simulink library "SingleWorkstationModelLibrary"  (R2014a)
settings: Solver=ode45  StartTime=0.0  StopTime=10.0  RelTol=1e-3
undefined symbols (not defined in the file or in its folder): se_randomizeseeds
(part 3 of 3)

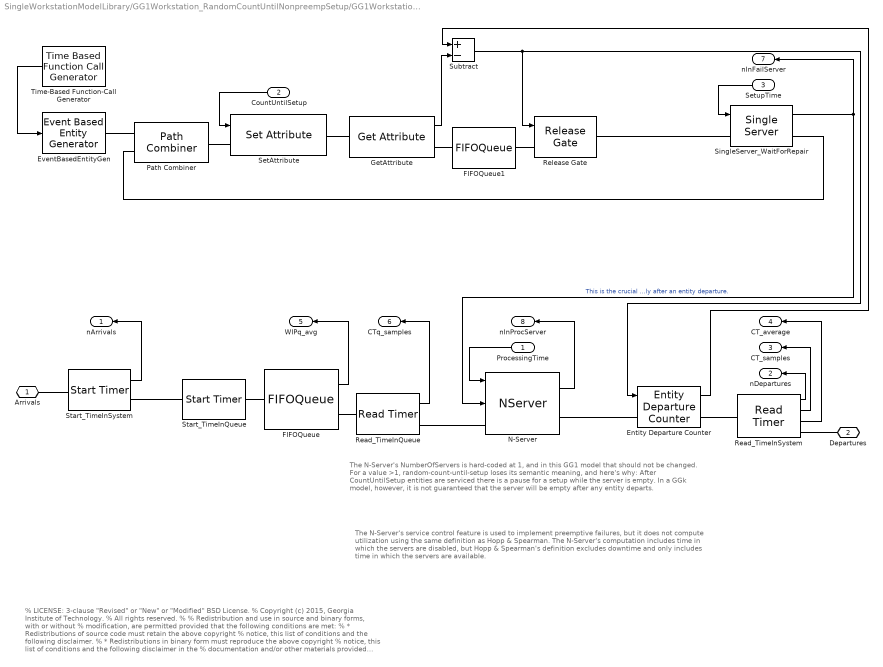
== system SingleWorkstationModelLibrary/GG1Workstation_RandomCountUntilNonpreempSetup/GG1Workstation_RandomCountUntilNonpreempSetup ==
  note: The N-Server's NumberOfServers is hard-coded at 1, and in this GG1 model that
      | should not be changed.  For a value >1, random-count-until-setup loses its semantic
      | meaning, and here's why:  After CountUntilSetup entities are serviced there is a pause
      | for a setup while the server is empty.  In a GGk model, however, it is not guaranteed
      | that the server will be empty after any entity departs.
  note: The N-Server's service control feature is used to implement preemptive failures,
      | but it does not compute utilization using the same definition as Hopp & Spearman.
      | The N-Server's computation includes time in which the servers are disabled, but
      | Hopp & Spearman's definition excludes downtime and only includes time in which
      | the servers are available.
  note: % LICENSE: 3-clause "Revised" or "New" or "Modified" BSD License.
      | % Copyright (c) 2015, Georgia Institute of Technology.
      | % All rights reserved.
      | %
      | % Redistribution and use in source and binary forms, with or without
      | % modification, are permitted provided that the following conditions are met:
      | % * Redistributions of source code must retain the above copyright
      | % notice, this list of conditions and the following disclaimer.
      | % * Redistributions in binary form must reproduce the above copyright
      | % notice, this list of conditions and the following disclaimer in the
      | % documentation and/or other materials provided with the distribution.
      | % * Neither the name of the Georgia Institute of Technology nor the
      | % names of its contributors may be used to endorse or promote products
      | % derived from this software without specific prior written permission.
      | %
      | % THIS SOFTWARE IS PROVIDED BY THE COPYRIGHT HOLDERS AND CONTRIBUTORS "AS IS" AND
      | % ANY EXPRESS OR IMPLIED WARRANTIES, INCLUDING, BUT NOT LIMITED TO, THE IMPLIED
      | % WARRANTIES OF MERCHANTABILITY AND FITNESS FOR A PARTICULAR PURPOSE ARE
      | % DISCLAIMED. IN NO EVENT SHALL THE GEORGIA INSTITUTE OF TECHNOLOGY BE LIABLE FOR
      | % ANY DIRECT, INDIRECT, INCIDENTAL, SPECIAL, EXEMPLARY, OR CONSEQUENTIAL DAMAGES
      | % (INCLUDING, BUT NOT LIMITED TO, PROCUREMENT OF SUBSTITUTE GOODS OR SERVICES;
      | % LOSS OF USE, DATA, OR PROFITS; OR BUSINESS INTERRUPTION) HOWEVER CAUSED AND
      | % ON ANY THEORY OF LIABILITY, WHETHER IN CONTRACT, STRICT LIABILITY, OR TORT
      | % (INCLUDING NEGLIGENCE OR OTHERWISE) ARISING IN ANY WAY OUT OF THE USE OF THIS
      | % SOFTWARE, EVEN IF ADVISED OF THE POSSIBILITY OF SUCH DAMAGE.
  ProcessingTime : Inport
  CountUntilSetup : Inport  Port=2
  SetupTime : Inport  Port=3
  Entity Departure Counter : EntityDepartureCounter  NumberDepartedToSignal=on  NumberDepartedToAttribute=off  CounterResetTypeOption=Trigger from port tr
  EventBasedEntityGen : EventBasedEntityGenerator  GenerateEntitiesUpon=Function call from port fcn
  FIFOQueue : FIFOQueue  Capacity=Capacity  StatAverageQueueLength=on
      settings: OutputPortMap=o3
  FIFOQueue1 : FIFOQueue  Capacity=Inf
  GetAttribute : GetAttribute  AttributeName=CountUntilSetup  EvaluatedDefaultAttributeValue={ []}
      settings: OutputPortMap=o1
  N-Server : NServer  NumberOfServers=1  ServiceTimeFrom=Signal port t  AllowServiceControl=on  BlockWhileSignalOn=on  StatNumberInBlock=on
      settings: InputPortMap=u0,u1  OutputPortMap=o1
  Path Combiner : PathCombiner  NumberInputPorts=2
  Read_TimeInQueue : ReadTimer  TimerTag=TimeInQueue  StatTimeElapsed=on
      settings: OutputPortMap=o2
  Read_TimeInSystem : ReadTimer  TimerTag=TimeInSystem  StatNumberDeparted=on  StatTimeElapsed=on  StatAverageTimeElapsed=on
      settings: OutputPortMap=o0,o2,o3
  Release Gate : ReleaseGate  OpenGateUpon=Trigger from port tr
  SetAttribute : SetAttribute  AttributeName=CountUntilSetup  AttributeFrom=Signal port  EvaluatedAttributeValue={ []}
  SingleServer_WaitForRepair : SingleServer  ServiceTimeFrom=Signal port t  AttributeName=SetupTime  StatNumberInBlock=on
      settings: OutputPortMap=o1
  Start_TimeInQueue : StartTimer  TimerTag=TimeInQueue  TimerStartedOption=Restart
  Start_TimeInSystem : StartTimer  TimerTag=TimeInSystem  TimerStartedOption=Restart  StatNumberDeparted=on
  Subtract : Sum  Inputs=+-
  Time-Based Function-Call Generator : TimeBasedFunctionCallGenerator  EventGenerationMode=Only at simulation start
  Arrivals : PMIOPort  Port=1  Side=Left
  Departures : PMIOPort  Port=2  Side=Right
  nArrivals : Outport
  nDepartures : Outport  Port=2
  CT_samples : Outport  Port=3
  CT_average : Outport  Port=4
  WIPq_avg : Outport  Port=5
  CTq_samples : Outport  Port=6
  nInFailServer : Outport  Port=7
  nInProcServer : Outport  Port=8
  wires:
  Read_TimeInSystem/2 -> CT_samples/1
  Read_TimeInQueue/1 -> CTq_samples/1
  FIFOQueue/1 -> WIPq_avg/1
  Start_TimeInSystem/1 -> nArrivals/1
  Read_TimeInSystem/1 -> nDepartures/1
  ProcessingTime/1 -> N-Server/1
  Read_TimeInSystem/3 -> CT_average/1
  Time-Based Function-Call Generator/1 -> EventBasedEntityGen/1
  CountUntilSetup/1 -> SetAttribute/1
  Subtract/1 -> Release Gate/1, Entity Departure Counter/1
  GetAttribute/1 -> Subtract/2
  Entity Departure Counter/1 -> Subtract/1
  SingleServer_WaitForRepair/1 -> nInFailServer/1, N-Server/2  "This is the crucial blocking signal - when > 0 the N-Server will be preemptively disabled. Non-preemption in this model is an approximation, because disabling of the N-Server  should follow shortly after an entity departure."
  N-Server/1 -> nInProcServer/1
  SetupTime/1 -> SingleServer_WaitForRepair/1
  connections:
  Arrivals/RConn1 -- Start_TimeInSystem/LConn1
  FIFOQueue/RConn1 -- Read_TimeInQueue/LConn1
  Start_TimeInSystem/RConn1 -- Start_TimeInQueue/LConn1
  Read_TimeInSystem/RConn1 -- Departures/RConn1
  Read_TimeInQueue/RConn1 -- N-Server/LConn1
  Start_TimeInQueue/RConn1 -- FIFOQueue/LConn1
  Path Combiner/RConn1 -- SetAttribute/LConn1
  EventBasedEntityGen/RConn1 -- Path Combiner/LConn1
  SingleServer_WaitForRepair/RConn1 -- Path Combiner/LConn2
  N-Server/RConn1 -- Entity Departure Counter/LConn1
  Entity Departure Counter/RConn1 -- Read_TimeInSystem/LConn1
  FIFOQueue1/LConn1 -- GetAttribute/RConn1
  Release Gate/RConn1 -- SingleServer_WaitForRepair/LConn1
  FIFOQueue1/RConn1 -- Release Gate/LConn1
  SetAttribute/RConn1 -- GetAttribute/LConn1

== system SingleWorkstationModelLibrary/GGkWorkstation/ComputeTH ==
  CurrentTime : Inport
  nDepartures : Inport  Port=2
  Derivative : Derivative
  Divide1 : Product  Inputs=/*
  Event to Timed Signal1 : EventToTimedSignal
  TH_average : Outport
  TH_samples : Outport  Port=2
  wires:
  CurrentTime/1 -> Divide1/1
  Event to Timed Signal1/1 -> Derivative/1, Divide1/2
  Divide1/1 -> TH_average/1
  Derivative/1 -> TH_samples/1
  nDepartures/1 -> Event to Timed Signal1/1

== system SingleWorkstationModelLibrary/GGkWorkstation/ComputeWIP ==
  nArrivals : Inport
  nDepartures : Inport  Port=2
  CurrentTime : Inport  Port=3
  Divide : Product  Inputs=*/
  Event to Timed Signal : EventToTimedSignal
  Integrator : Integrator
  Subtract : Sum  Inputs=+-
  WIP_samples : Outport
  WIP_average : Outport  Port=2
  wires:
  Subtract/1 -> WIP_samples/1, Event to Timed Signal/1
  Event to Timed Signal/1 -> Integrator/1
  Divide/1 -> WIP_average/1
  Integrator/1 -> Divide/1
  nArrivals/1 -> Subtract/1
  nDepartures/1 -> Subtract/2
  CurrentTime/1 -> Divide/2

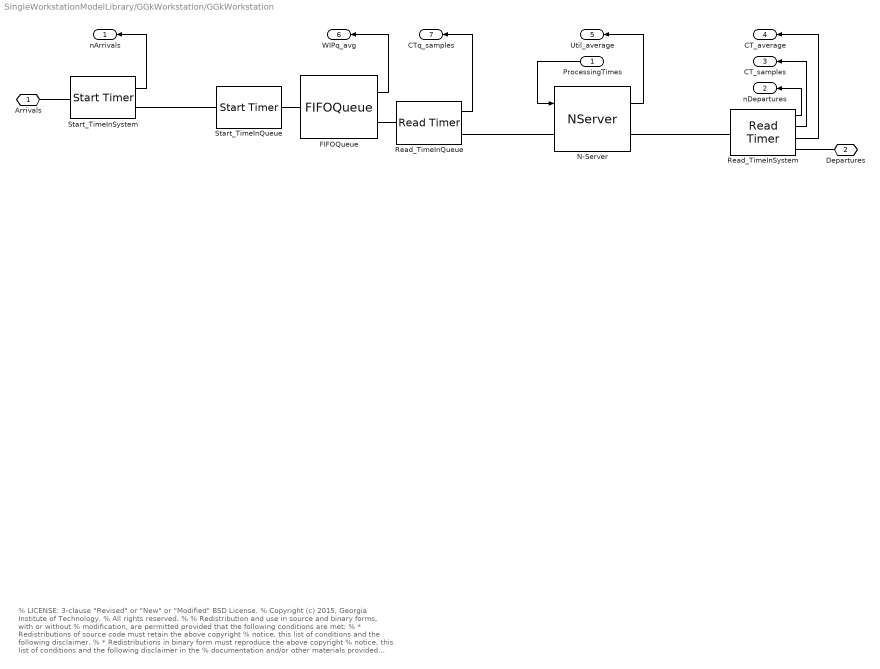
== system SingleWorkstationModelLibrary/GGkWorkstation/GGkWorkstation ==
  note: % LICENSE: 3-clause "Revised" or "New" or "Modified" BSD License.
      | % Copyright (c) 2015, Georgia Institute of Technology.
      | % All rights reserved.
      | %
      | % Redistribution and use in source and binary forms, with or without
      | % modification, are permitted provided that the following conditions are met:
      | % * Redistributions of source code must retain the above copyright
      | % notice, this list of conditions and the following disclaimer.
      | % * Redistributions in binary form must reproduce the above copyright
      | % notice, this list of conditions and the following disclaimer in the
      | % documentation and/or other materials provided with the distribution.
      | % * Neither the name of the Georgia Institute of Technology nor the
      | % names of its contributors may be used to endorse or promote products
      | % derived from this software without specific prior written permission.
      | %
      | % THIS SOFTWARE IS PROVIDED BY THE COPYRIGHT HOLDERS AND CONTRIBUTORS "AS IS" AND
      | % ANY EXPRESS OR IMPLIED WARRANTIES, INCLUDING, BUT NOT LIMITED TO, THE IMPLIED
      | % WARRANTIES OF MERCHANTABILITY AND FITNESS FOR A PARTICULAR PURPOSE ARE
      | % DISCLAIMED. IN NO EVENT SHALL THE GEORGIA INSTITUTE OF TECHNOLOGY BE LIABLE FOR
      | % ANY DIRECT, INDIRECT, INCIDENTAL, SPECIAL, EXEMPLARY, OR CONSEQUENTIAL DAMAGES
      | % (INCLUDING, BUT NOT LIMITED TO, PROCUREMENT OF SUBSTITUTE GOODS OR SERVICES;
      | % LOSS OF USE, DATA, OR PROFITS; OR BUSINESS INTERRUPTION) HOWEVER CAUSED AND
      | % ON ANY THEORY OF LIABILITY, WHETHER IN CONTRACT, STRICT LIABILITY, OR TORT
      | % (INCLUDING NEGLIGENCE OR OTHERWISE) ARISING IN ANY WAY OUT OF THE USE OF THIS
      | % SOFTWARE, EVEN IF ADVISED OF THE POSSIBILITY OF SUCH DAMAGE.
  ProcessingTimes : Inport
  FIFOQueue : FIFOQueue  Capacity=Capacity  StatAverageQueueLength=on
      settings: OutputPortMap=o3
  N-Server : NServer  NumberOfServers=NumberOfServers  ServiceTimeFrom=Signal port t  StatUtilization=on
      settings: OutputPortMap=o5
  Read_TimeInQueue : ReadTimer  TimerTag=TimeInQueue  StatTimeElapsed=on
      settings: OutputPortMap=o2
  Read_TimeInSystem : ReadTimer  TimerTag=TimeInSystem  StatNumberDeparted=on  StatTimeElapsed=on  StatAverageTimeElapsed=on
      settings: OutputPortMap=o0,o2,o3
  Start_TimeInQueue : StartTimer  TimerTag=TimeInQueue  TimerStartedOption=Restart
  Start_TimeInSystem : StartTimer  TimerTag=TimeInSystem  TimerStartedOption=Restart  StatNumberDeparted=on
  Arrivals : PMIOPort  Port=1  Side=Left
  Departures : PMIOPort  Port=2  Side=Right
  nArrivals : Outport
  nDepartures : Outport  Port=2
  CT_samples : Outport  Port=3
  CT_average : Outport  Port=4
  Util_average : Outport  Port=5
  WIPq_avg : Outport  Port=6
  CTq_samples : Outport  Port=7
  wires:
  Read_TimeInSystem/2 -> CT_samples/1
  N-Server/1 -> Util_average/1
  Read_TimeInQueue/1 -> CTq_samples/1
  FIFOQueue/1 -> WIPq_avg/1
  Start_TimeInSystem/1 -> nArrivals/1
  Read_TimeInSystem/1 -> nDepartures/1
  ProcessingTimes/1 -> N-Server/1
  Read_TimeInSystem/3 -> CT_average/1
  connections:
  Arrivals/RConn1 -- Start_TimeInSystem/LConn1
  N-Server/RConn1 -- Read_TimeInSystem/LConn1
  FIFOQueue/RConn1 -- Read_TimeInQueue/LConn1
  Start_TimeInSystem/RConn1 -- Start_TimeInQueue/LConn1
  Read_TimeInSystem/RConn1 -- Departures/RConn1
  Read_TimeInQueue/RConn1 -- N-Server/LConn1
  Start_TimeInQueue/RConn1 -- FIFOQueue/LConn1

== system SingleWorkstationModelLibrary/GGkWorkstation_MakeAndMoveBatches_Parallel/ComputeTH ==
  CurrentTime : Inport
  nDepartures : Inport  Port=2
  Derivative : Derivative
  Divide1 : Product  Inputs=/*
  Event to Timed Signal1 : EventToTimedSignal
  TH_average : Outport
  TH_samples : Outport  Port=2
  wires:
  CurrentTime/1 -> Divide1/1
  Event to Timed Signal1/1 -> Derivative/1, Divide1/2
  Divide1/1 -> TH_average/1
  Derivative/1 -> TH_samples/1
  nDepartures/1 -> Event to Timed Signal1/1

== system SingleWorkstationModelLibrary/GGkWorkstation_MakeAndMoveBatches_Parallel/ComputeWIP ==
  nArrivals : Inport
  nDepartures : Inport  Port=2
  CurrentTime : Inport  Port=3
  Divide : Product  Inputs=*/
  Event to Timed Signal : EventToTimedSignal
  Integrator : Integrator
  Subtract : Sum  Inputs=+-
  WIP_samples : Outport
  WIP_average : Outport  Port=2
  wires:
  Subtract/1 -> WIP_samples/1, Event to Timed Signal/1
  Event to Timed Signal/1 -> Integrator/1
  Divide/1 -> WIP_average/1
  Integrator/1 -> Divide/1
  nArrivals/1 -> Subtract/1
  nDepartures/1 -> Subtract/2
  CurrentTime/1 -> Divide/2

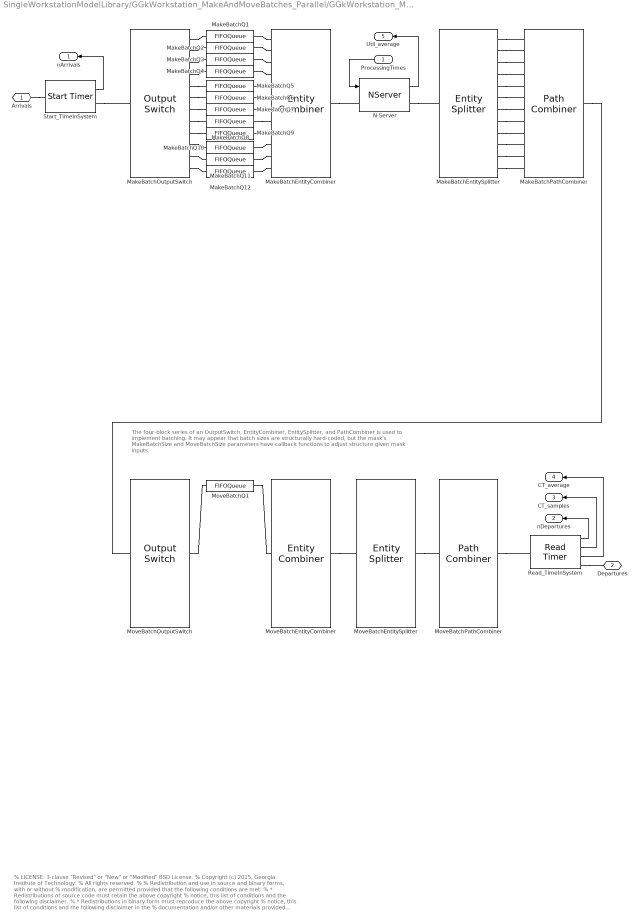
== system SingleWorkstationModelLibrary/GGkWorkstation_MakeAndMoveBatches_Parallel/GGkWorkstation_MakeAndMoveBatches_Parallel ==
  note: The four-block series of an OutputSwitch, EntityCombiner, EntitySplitter, and PathCombiner is used
      | to implement batching. It may appear that batch sizes are structurally hard-coded, but the mask's
      | MakeBatchSize and MoveBatchSize parameters have callback functions to adjust structure given
      | mask inputs.
  note: % LICENSE: 3-clause "Revised" or "New" or "Modified" BSD License.
      | % Copyright (c) 2015, Georgia Institute of Technology.
      | % All rights reserved.
      | %
      | % Redistribution and use in source and binary forms, with or without
      | % modification, are permitted provided that the following conditions are met:
      | % * Redistributions of source code must retain the above copyright
      | % notice, this list of conditions and the following disclaimer.
      | % * Redistributions in binary form must reproduce the above copyright
      | % notice, this list of conditions and the following disclaimer in the
      | % documentation and/or other materials provided with the distribution.
      | % * Neither the name of the Georgia Institute of Technology nor the
      | % names of its contributors may be used to endorse or promote products
      | % derived from this software without specific prior written permission.
      | %
      | % THIS SOFTWARE IS PROVIDED BY THE COPYRIGHT HOLDERS AND CONTRIBUTORS "AS IS" AND
      | % ANY EXPRESS OR IMPLIED WARRANTIES, INCLUDING, BUT NOT LIMITED TO, THE IMPLIED
      | % WARRANTIES OF MERCHANTABILITY AND FITNESS FOR A PARTICULAR PURPOSE ARE
      | % DISCLAIMED. IN NO EVENT SHALL THE GEORGIA INSTITUTE OF TECHNOLOGY BE LIABLE FOR
      | % ANY DIRECT, INDIRECT, INCIDENTAL, SPECIAL, EXEMPLARY, OR CONSEQUENTIAL DAMAGES
      | % (INCLUDING, BUT NOT LIMITED TO, PROCUREMENT OF SUBSTITUTE GOODS OR SERVICES;
      | % LOSS OF USE, DATA, OR PROFITS; OR BUSINESS INTERRUPTION) HOWEVER CAUSED AND
      | % ON ANY THEORY OF LIABILITY, WHETHER IN CONTRACT, STRICT LIABILITY, OR TORT
      | % (INCLUDING NEGLIGENCE OR OTHERWISE) ARISING IN ANY WAY OUT OF THE USE OF THIS
      | % SOFTWARE, EVEN IF ADVISED OF THE POSSIBILITY OF SUCH DAMAGE.
  ProcessingTimes : Inport
  MakeBatchEntityCombiner : EntityCombiner  NumberInputPorts=12  AttributeAccessibility=off  TimerAccessibility=off
  MakeBatchEntitySplitter : EntitySplitter  NumberOutputPorts=12
  MakeBatchOutputSwitch : OutputSwitch  NumberOutputPorts=12  SwitchingCriterion=Round robin
  MakeBatchPathCombiner : PathCombiner  NumberInputPorts=12
  MakeBatchQ{1..12} (12 alike) : FIFOQueue  Capacity=Inf
  MoveBatchEntityCombiner : EntityCombiner  NumberInputPorts=1  AttributeAccessibility=off  TimerAccessibility=off
  MoveBatchEntitySplitter : EntitySplitter  NumberOutputPorts=1
  MoveBatchOutputSwitch : OutputSwitch  NumberOutputPorts=1  SwitchingCriterion=Round robin
  MoveBatchPathCombiner : PathCombiner  NumberInputPorts=1
  MoveBatchQ1 : FIFOQueue  Capacity=Inf
  N-Server : NServer  NumberOfServers=NumberOfServers  ServiceTimeFrom=Signal port t  StatUtilization=on
      settings: OutputPortMap=o5
  Read_TimeInSystem : ReadTimer  TimerTag=TimeInSystem  StatNumberDeparted=on  StatTimeElapsed=on  StatAverageTimeElapsed=on
      settings: OutputPortMap=o0,o2,o3
  Start_TimeInSystem : StartTimer  TimerTag=TimeInSystem  TimerStartedOption=Restart  StatNumberDeparted=on
  Arrivals : PMIOPort  Port=1  Side=Left
  Departures : PMIOPort  Port=2  Side=Right
  nArrivals : Outport
  nDepartures : Outport  Port=2
  CT_samples : Outport  Port=3
  CT_average : Outport  Port=4
  Util_average : Outport  Port=5
  wires:
  Start_TimeInSystem/1 -> nArrivals/1
  Read_TimeInSystem/1 -> nDepartures/1
  Read_TimeInSystem/2 -> CT_samples/1
  N-Server/1 -> Util_average/1
  Read_TimeInSystem/3 -> CT_average/1
  ProcessingTimes/1 -> N-Server/1
  connections:
  MoveBatchEntityCombiner/RConn1 -- MoveBatchEntitySplitter/LConn1
  Read_TimeInSystem/RConn1 -- Departures/RConn1
  Arrivals/RConn1 -- Start_TimeInSystem/LConn1
  Start_TimeInSystem/RConn1 -- MakeBatchOutputSwitch/LConn1
  MakeBatchEntityCombiner/RConn1 -- N-Server/LConn1
  N-Server/RConn1 -- MakeBatchEntitySplitter/LConn1
  MakeBatchPathCombiner/RConn1 -- MoveBatchOutputSwitch/LConn1
  MoveBatchPathCombiner/RConn1 -- Read_TimeInSystem/LConn1
  MakeBatchOutputSwitch/RConn1 -- MakeBatchQ1/LConn1
  MakeBatchQ1/RConn1 -- MakeBatchEntityCombiner/LConn1
  MakeBatchOutputSwitch/RConn2 -- MakeBatchQ2/LConn1
  MakeBatchQ2/RConn1 -- MakeBatchEntityCombiner/LConn2
  MakeBatchOutputSwitch/RConn3 -- MakeBatchQ3/LConn1
  MakeBatchQ3/RConn1 -- MakeBatchEntityCombiner/LConn3
  MakeBatchOutputSwitch/RConn4 -- MakeBatchQ4/LConn1
  MakeBatchQ4/RConn1 -- MakeBatchEntityCombiner/LConn4
  MakeBatchOutputSwitch/RConn5 -- MakeBatchQ5/LConn1
  MakeBatchQ5/RConn1 -- MakeBatchEntityCombiner/LConn5
  MakeBatchOutputSwitch/RConn6 -- MakeBatchQ6/LConn1
  MakeBatchQ6/RConn1 -- MakeBatchEntityCombiner/LConn6
  MakeBatchOutputSwitch/RConn7 -- MakeBatchQ7/LConn1
  MakeBatchQ7/RConn1 -- MakeBatchEntityCombiner/LConn7
  MakeBatchOutputSwitch/RConn8 -- MakeBatchQ8/LConn1
  MakeBatchQ8/RConn1 -- MakeBatchEntityCombiner/LConn8
  MakeBatchOutputSwitch/RConn9 -- MakeBatchQ9/LConn1
  MakeBatchQ9/RConn1 -- MakeBatchEntityCombiner/LConn9
  MakeBatchOutputSwitch/RConn10 -- MakeBatchQ10/LConn1
  MakeBatchQ10/RConn1 -- MakeBatchEntityCombiner/LConn10
  MakeBatchOutputSwitch/RConn11 -- MakeBatchQ11/LConn1
  MakeBatchQ11/RConn1 -- MakeBatchEntityCombiner/LConn11
  MakeBatchOutputSwitch/RConn12 -- MakeBatchQ12/LConn1
  MakeBatchQ12/RConn1 -- MakeBatchEntityCombiner/LConn12
  MakeBatchEntitySplitter/RConn1 -- MakeBatchPathCombiner/LConn1
  MakeBatchEntitySplitter/RConn2 -- MakeBatchPathCombiner/LConn2
  MakeBatchEntitySplitter/RConn3 -- MakeBatchPathCombiner/LConn3
  MakeBatchEntitySplitter/RConn4 -- MakeBatchPathCombiner/LConn4
  MakeBatchEntitySplitter/RConn5 -- MakeBatchPathCombiner/LConn5
  MakeBatchEntitySplitter/RConn6 -- MakeBatchPathCombiner/LConn6
  MakeBatchEntitySplitter/RConn7 -- MakeBatchPathCombiner/LConn7
  MakeBatchEntitySplitter/RConn8 -- MakeBatchPathCombiner/LConn8
  MakeBatchEntitySplitter/RConn9 -- MakeBatchPathCombiner/LConn9
  MakeBatchEntitySplitter/RConn10 -- MakeBatchPathCombiner/LConn10
  MakeBatchEntitySplitter/RConn11 -- MakeBatchPathCombiner/LConn11
  MakeBatchEntitySplitter/RConn12 -- MakeBatchPathCombiner/LConn12
  MoveBatchOutputSwitch/RConn1 -- MoveBatchQ1/LConn1
  MoveBatchQ1/RConn1 -- MoveBatchEntityCombiner/LConn1
  MoveBatchEntitySplitter/RConn1 -- MoveBatchPathCombiner/LConn1
